simulink model "Offline_DataImport_AND_SCGAnalysis"  (R2020b)
settings: Solver=FixedStepDiscrete  StartTime=0.0  StopTime=param_sim_time  FixedStep=1/fs  MaxStep=1/fs  RelTol=1e-3
undefined symbols (not defined in the file): analyses, fs, param_tot_samples
libraries: dspstat3 x1
settings Model: PacingRate=100  Creator=rcord  LastModifiedBy=Rafael
settings SolverCC: ZeroCrossControl=DisableAll
settings DataIOCC: ExternalInput=[t, signals.scg.preprocessed_x, signals.scg.preprocessed_y, signals.scg.preprocessed_z]  LoadExternalInput=on  SignalLogging=off  DSMLogging=off  SaveTime=off  ReturnWorkspaceOutputs=off  TimeSaveName=t_preprocessing  OutputSaveName=out_SCGAnalysis  LoggingIntervals=[-inf,inf]
settings SFSimCC: CustomCodeUndefinedFunction=UseInterfaceOnly

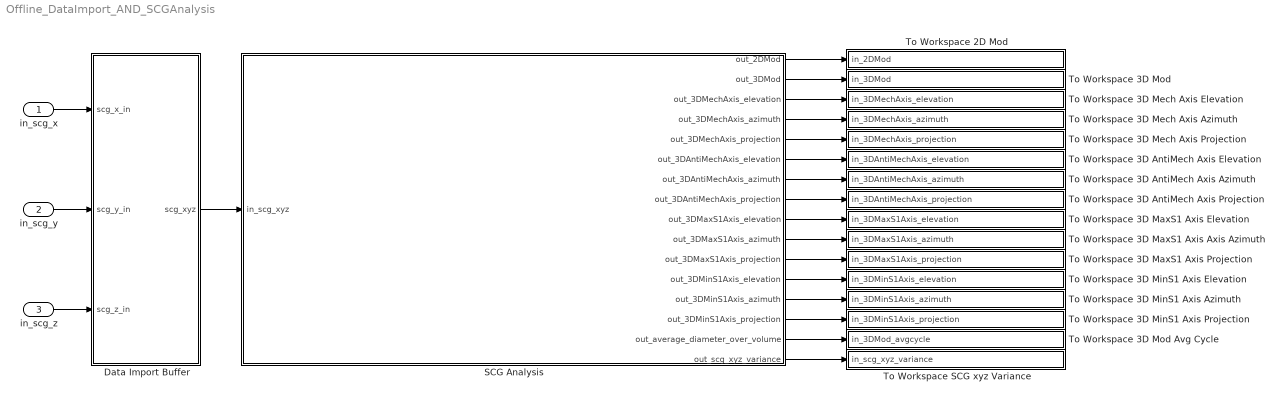
== system Offline_DataImport_AND_SCGAnalysis ==
  in_scg_x : Inport  SampleTime=1/fs
  in_scg_y : Inport  Port=2  SampleTime=1/fs
  in_scg_z : Inport  Port=3  SampleTime=1/fs
  Data Import Buffer : Subsystem
  SCG Analysis : Subsystem
      mask Display: image('C:\Users\Rafael\Dropbox\Post-Doc Research\SCG Analysis.png'); % Use "Edit Image" on toolstrip to change.
  To Workspace 2D Mod : Subsystem
      mask Display: disp('out_scg_analysis_2DMod')
  To Workspace 3D AntiMech Axis Azimuth : Subsystem
      mask Display: disp('out_scg_analysis_3DAntiMechAxis_azimuth')
  To Workspace 3D AntiMech Axis Elevation : Subsystem
      mask Display: disp('out_scg_analysis_3DAntiMechAxis_elevation')
  To Workspace 3D AntiMech Axis Projection : Subsystem
      mask Display: disp('out_scg_analysis_3DAntiMechAxis_projection')
  To Workspace 3D MaxS1 Axis Axis Azimuth : Subsystem
      mask Display: disp('out_scg_analysis_3DMaxS1Axis_azimuth')
  To Workspace 3D MaxS1 Axis Elevation : Subsystem
      mask Display: disp('out_scg_analysis_3DMaxS1Axis_elevation')
  To Workspace 3D MaxS1 Axis Projection : Subsystem
      mask Display: disp('out_scg_analysis_3DMaxS1Axis_projection')
  To Workspace 3D Mech Axis Azimuth : Subsystem
      mask Display: disp('out_scg_analysis_3DMechAxis_azimuth')
  To Workspace 3D Mech Axis Elevation : Subsystem
      mask Display: disp('out_scg_analysis_3DMechAxis_elevation')
  To Workspace 3D Mech Axis Projection : Subsystem
      mask Display: disp('out_scg_analysis_3DMechAxis_projection')
  To Workspace 3D MinS1 Axis Azimuth : Subsystem
      mask Display: disp('out_scg_analysis_3DMinS1Axis_azimuth')
  To Workspace 3D MinS1 Axis Elevation : Subsystem
      mask Display: disp('out_scg_analysis_3DMinS1Axis_elevation')
  To Workspace 3D MinS1 Axis Projection : Subsystem
      mask Display: disp('out_scg_analysis_3DMinS1Axis_projection')
  To Workspace 3D Mod : Subsystem
      mask Display: disp('out_scg_analysis_3DMod')
  To Workspace 3D Mod Avg Cycle : Subsystem
      mask Display: disp('out_scg_analysis_3DMod_avgcycle')
  To Workspace SCG xyz Variance : Subsystem
      mask Display: disp('out_scg_analysis_scg_xyz_variance')
  wires:
  in_scg_x/1 -> Data Import Buffer/1(scg_x_in)
  in_scg_y/1 -> Data Import Buffer/2(scg_y_in)
  in_scg_z/1 -> Data Import Buffer/3(scg_z_in)
  Data Import Buffer/1(scg_xyz) -> SCG Analysis/1(in_scg_xyz)
  SCG Analysis/16(out_scg_xyz_variance) -> To Workspace SCG xyz Variance/1(in_scg_xyz_variance)
  SCG Analysis/2(out_3DMod) -> To Workspace 3D Mod/1(in_3DMod)
  SCG Analysis/15(out_average_diameter_over_volume) -> To Workspace 3D Mod Avg Cycle/1(in_3DMod_avgcycle)
  SCG Analysis/1(out_2DMod) -> To Workspace 2D Mod/1(in_2DMod)
  SCG Analysis/3(out_3DMechAxis_elevation) -> To Workspace 3D Mech Axis Elevation/1(in_3DMechAxis_elevation)
  SCG Analysis/4(out_3DMechAxis_azimuth) -> To Workspace 3D Mech Axis Azimuth/1(in_3DMechAxis_azimuth)
  SCG Analysis/5(out_3DMechAxis_projection) -> To Workspace 3D Mech Axis Projection/1(in_3DMechAxis_projection)
  SCG Analysis/6(out_3DAntiMechAxis_elevation) -> To Workspace 3D AntiMech Axis Elevation/1(in_3DAntiMechAxis_elevation)
  SCG Analysis/7(out_3DAntiMechAxis_azimuth) -> To Workspace 3D AntiMech Axis Azimuth/1(in_3DAntiMechAxis_azimuth)
  SCG Analysis/8(out_3DAntiMechAxis_projection) -> To Workspace 3D AntiMech Axis Projection/1(in_3DAntiMechAxis_projection)
  SCG Analysis/9(out_3DMaxS1Axis_elevation) -> To Workspace 3D MaxS1 Axis Elevation/1(in_3DMaxS1Axis_elevation)
  SCG Analysis/10(out_3DMaxS1Axis_azimuth) -> To Workspace 3D MaxS1 Axis Axis Azimuth/1(in_3DMaxS1Axis_azimuth)
  SCG Analysis/11(out_3DMaxS1Axis_projection) -> To Workspace 3D MaxS1 Axis Projection/1(in_3DMaxS1Axis_projection)
  SCG Analysis/12(out_3DMinS1Axis_elevation) -> To Workspace 3D MinS1 Axis Elevation/1(in_3DMinS1Axis_elevation)
  SCG Analysis/13(out_3DMinS1Axis_azimuth) -> To Workspace 3D MinS1 Axis Azimuth/1(in_3DMinS1Axis_azimuth)
  SCG Analysis/14(out_3DMinS1Axis_projection) -> To Workspace 3D MinS1 Axis Projection/1(in_3DMinS1Axis_projection)

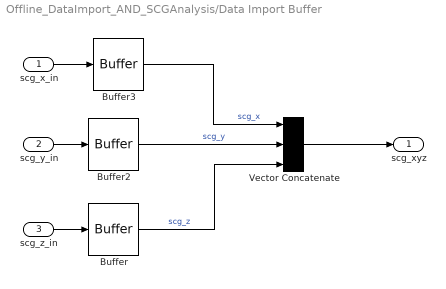
== system Offline_DataImport_AND_SCGAnalysis/Data Import Buffer ==
  scg_x_in : Inport
  scg_y_in : Inport  Port=2
  scg_z_in : Inport  Port=3
  Buffer : Buffer  N=param_tot_samples  OutputFrames=off
  Buffer2 : Buffer  N=param_tot_samples  OutputFrames=off
  Buffer3 : Buffer  N=param_tot_samples  OutputFrames=off
  Vector Concatenate : Concatenate  NumInputs=3  Mode=Multidimensional array  ConcatenateDimension=2
  scg_xyz : Outport  VectorParamsAs1DForOutWhenUnconnected=off
  wires:
  Buffer/1 -> Vector Concatenate/3  "scg_z"
  Buffer3/1 -> Vector Concatenate/1  "scg_x"
  scg_x_in/1 -> Buffer3/1
  Vector Concatenate/1 -> scg_xyz/1
  Buffer2/1 -> Vector Concatenate/2  "scg_y"
  scg_z_in/1 -> Buffer/1
  scg_y_in/1 -> Buffer2/1

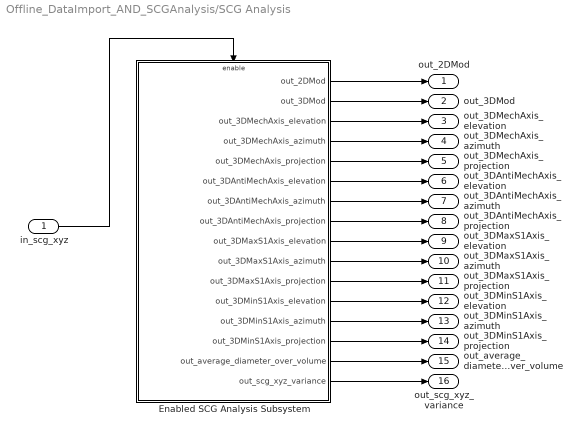
== system Offline_DataImport_AND_SCGAnalysis/SCG Analysis ==
  in_scg_xyz : Inport
  Enabled SCG Analysis Subsystem : Subsystem  TreatAsAtomicUnit=on
  out_2DMod : Outport  VectorParamsAs1DForOutWhenUnconnected=off
  out_3DMod : Outport  Port=2  VectorParamsAs1DForOutWhenUnconnected=off
  out_3DMechAxis_elevation : Outport  Port=3  VectorParamsAs1DForOutWhenUnconnected=off
  out_3DMechAxis_azimuth : Outport  Port=4  VectorParamsAs1DForOutWhenUnconnected=off
  out_3DMechAxis_projection : Outport  Port=5  VectorParamsAs1DForOutWhenUnconnected=off
  out_3DAntiMechAxis_elevation : Outport  Port=6  VectorParamsAs1DForOutWhenUnconnected=off
  out_3DAntiMechAxis_azimuth : Outport  Port=7  VectorParamsAs1DForOutWhenUnconnected=off
  out_3DAntiMechAxis_projection : Outport  Port=8  VectorParamsAs1DForOutWhenUnconnected=off
  out_3DMaxS1Axis_elevation : Outport  Port=9  VectorParamsAs1DForOutWhenUnconnected=off
  out_3DMaxS1Axis_azimuth : Outport  Port=10  VectorParamsAs1DForOutWhenUnconnected=off
  out_3DMaxS1Axis_projection : Outport  Port=11  VectorParamsAs1DForOutWhenUnconnected=off
  out_3DMinS1Axis_elevation : Outport  Port=12  VectorParamsAs1DForOutWhenUnconnected=off
  out_3DMinS1Axis_azimuth : Outport  Port=13  VectorParamsAs1DForOutWhenUnconnected=off
  out_3DMinS1Axis_projection : Outport  Port=14  VectorParamsAs1DForOutWhenUnconnected=off
  out_average_diameter_over_volume : Outport  Port=15  VectorParamsAs1DForOutWhenUnconnected=off
  out_scg_xyz_variance : Outport  Port=16  VectorParamsAs1DForOutWhenUnconnected=off
  wires:
  in_scg_xyz/1 -> Enabled SCG Analysis Subsystem/Enable
  Enabled SCG Analysis Subsystem/16(out_scg_xyz_variance) -> out_scg_xyz_variance/1
  Enabled SCG Analysis Subsystem/2(out_3DMod) -> out_3DMod/1
  Enabled SCG Analysis Subsystem/1(out_2DMod) -> out_2DMod/1
  Enabled SCG Analysis Subsystem/3(out_3DMechAxis_elevation) -> out_3DMechAxis_elevation/1
  Enabled SCG Analysis Subsystem/4(out_3DMechAxis_azimuth) -> out_3DMechAxis_azimuth/1
  Enabled SCG Analysis Subsystem/5(out_3DMechAxis_projection) -> out_3DMechAxis_projection/1
  Enabled SCG Analysis Subsystem/8(out_3DAntiMechAxis_projection) -> out_3DAntiMechAxis_projection/1
  Enabled SCG Analysis Subsystem/9(out_3DMaxS1Axis_elevation) -> out_3DMaxS1Axis_elevation/1
  Enabled SCG Analysis Subsystem/10(out_3DMaxS1Axis_azimuth) -> out_3DMaxS1Axis_azimuth/1
  Enabled SCG Analysis Subsystem/11(out_3DMaxS1Axis_projection) -> out_3DMaxS1Axis_projection/1
  Enabled SCG Analysis Subsystem/14(out_3DMinS1Axis_projection) -> out_3DMinS1Axis_projection/1
  Enabled SCG Analysis Subsystem/15(out_average_diameter_over_volume) -> out_average_diameter_over_volume/1
  Enabled SCG Analysis Subsystem/6(out_3DAntiMechAxis_elevation) -> out_3DAntiMechAxis_elevation/1
  Enabled SCG Analysis Subsystem/7(out_3DAntiMechAxis_azimuth) -> out_3DAntiMechAxis_azimuth/1
  Enabled SCG Analysis Subsystem/12(out_3DMinS1Axis_elevation) -> out_3DMinS1Axis_elevation/1
  Enabled SCG Analysis Subsystem/13(out_3DMinS1Axis_azimuth) -> out_3DMinS1Axis_azimuth/1

== system Offline_DataImport_AND_SCGAnalysis/To Workspace 2D Mod ==
  in_2DMod : Inport
  Enabled To Workspace 2DMod Subsystem : Subsystem  TreatAsAtomicUnit=on
  wires:
  in_2DMod/1 -> Enabled To Workspace 2DMod Subsystem/Enable

== system Offline_DataImport_AND_SCGAnalysis/To Workspace 3D AntiMech Axis Azimuth ==
  in_3DAntiMechAxis_azimuth : Inport
  Enabled To Workspace 3DAntiMechAxis Azimuth : Subsystem  TreatAsAtomicUnit=on
  wires:
  in_3DAntiMechAxis_azimuth/1 -> Enabled To Workspace 3DAntiMechAxis Azimuth/Enable

== system Offline_DataImport_AND_SCGAnalysis/To Workspace 3D AntiMech Axis Elevation ==
  in_3DAntiMechAxis_elevation : Inport
  Enabled To Workspace 3DAntiMechAxis Elevation : Subsystem  TreatAsAtomicUnit=on
  wires:
  in_3DAntiMechAxis_elevation/1 -> Enabled To Workspace 3DAntiMechAxis Elevation/Enable

== system Offline_DataImport_AND_SCGAnalysis/To Workspace 3D AntiMech Axis Projection ==
  in_3DAntiMechAxis_projection : Inport
  Enabled To Workspace 3DAntiMechAxis Projection : Subsystem  TreatAsAtomicUnit=on
  wires:
  in_3DAntiMechAxis_projection/1 -> Enabled To Workspace 3DAntiMechAxis Projection/Enable

== system Offline_DataImport_AND_SCGAnalysis/To Workspace 3D MaxS1 Axis Axis Azimuth ==
  in_3DMaxS1Axis_azimuth : Inport
  Enabled To Workspace 3DMaxS1Axis Azimuth : Subsystem  TreatAsAtomicUnit=on
  wires:
  in_3DMaxS1Axis_azimuth/1 -> Enabled To Workspace 3DMaxS1Axis Azimuth/Enable

== system Offline_DataImport_AND_SCGAnalysis/To Workspace 3D MaxS1 Axis Elevation ==
  in_3DMaxS1Axis_elevation : Inport
  Enabled To Workspace 3DMaxS1Axis Elevation : Subsystem  TreatAsAtomicUnit=on
  wires:
  in_3DMaxS1Axis_elevation/1 -> Enabled To Workspace 3DMaxS1Axis Elevation/Enable

== system Offline_DataImport_AND_SCGAnalysis/To Workspace 3D MaxS1 Axis Projection ==
  in_3DMaxS1Axis_projection : Inport
  Enabled To Workspace 3DMaxS1Axis Projection : Subsystem  TreatAsAtomicUnit=on
  wires:
  in_3DMaxS1Axis_projection/1 -> Enabled To Workspace 3DMaxS1Axis Projection/Enable

== system Offline_DataImport_AND_SCGAnalysis/To Workspace 3D Mech Axis Azimuth ==
  in_3DMechAxis_azimuth : Inport
  Enabled To Workspace 3DMechAxis Azimuth : Subsystem  TreatAsAtomicUnit=on
  wires:
  in_3DMechAxis_azimuth/1 -> Enabled To Workspace 3DMechAxis Azimuth/Enable

== system Offline_DataImport_AND_SCGAnalysis/To Workspace 3D Mech Axis Elevation ==
  in_3DMechAxis_elevation : Inport
  Enabled To Workspace 3DMechAxis Elevation : Subsystem  TreatAsAtomicUnit=on
  wires:
  in_3DMechAxis_elevation/1 -> Enabled To Workspace 3DMechAxis Elevation/Enable

== system Offline_DataImport_AND_SCGAnalysis/To Workspace 3D Mech Axis Projection ==
  in_3DMechAxis_projection : Inport
  Enabled To Workspace 3DMechAxis Projection : Subsystem  TreatAsAtomicUnit=on
  wires:
  in_3DMechAxis_projection/1 -> Enabled To Workspace 3DMechAxis Projection/Enable

== system Offline_DataImport_AND_SCGAnalysis/To Workspace 3D MinS1 Axis Azimuth ==
  in_3DMinS1Axis_azimuth : Inport
  Enabled To Workspace 3DMinS1Axis Azimuth : Subsystem  TreatAsAtomicUnit=on
  wires:
  in_3DMinS1Axis_azimuth/1 -> Enabled To Workspace 3DMinS1Axis Azimuth/Enable

== system Offline_DataImport_AND_SCGAnalysis/To Workspace 3D MinS1 Axis Elevation ==
  in_3DMinS1Axis_elevation : Inport
  Enabled To Workspace 3DMinS1Axis Elevation : Subsystem  TreatAsAtomicUnit=on
  wires:
  in_3DMinS1Axis_elevation/1 -> Enabled To Workspace 3DMinS1Axis Elevation/Enable

== system Offline_DataImport_AND_SCGAnalysis/To Workspace 3D MinS1 Axis Projection ==
  in_3DMinS1Axis_projection : Inport
  Enabled To Workspace 3DMinS1Axis Projection : Subsystem  TreatAsAtomicUnit=on
  wires:
  in_3DMinS1Axis_projection/1 -> Enabled To Workspace 3DMinS1Axis Projection/Enable

== system Offline_DataImport_AND_SCGAnalysis/To Workspace 3D Mod ==
  in_3DMod : Inport
  Enabled To Workspace 3DMod Subsystem : Subsystem  TreatAsAtomicUnit=on
  wires:
  in_3DMod/1 -> Enabled To Workspace 3DMod Subsystem/Enable

== system Offline_DataImport_AND_SCGAnalysis/To Workspace 3D Mod Avg Cycle ==
  in_3DMod_avgcycle : Inport
  Enabled To Workspace 3DMod Avg Cycle Subsystem : Subsystem  TreatAsAtomicUnit=on
  wires:
  in_3DMod_avgcycle/1 -> Enabled To Workspace 3DMod Avg Cycle Subsystem/Enable

== system Offline_DataImport_AND_SCGAnalysis/To Workspace SCG xyz Variance ==
  in_scg_xyz_variance : Inport
  Enabled To Workspace SCG xyz Variance Subsystem : Subsystem  TreatAsAtomicUnit=on
  wires:
  in_scg_xyz_variance/1 -> Enabled To Workspace SCG xyz Variance Subsystem/Enable

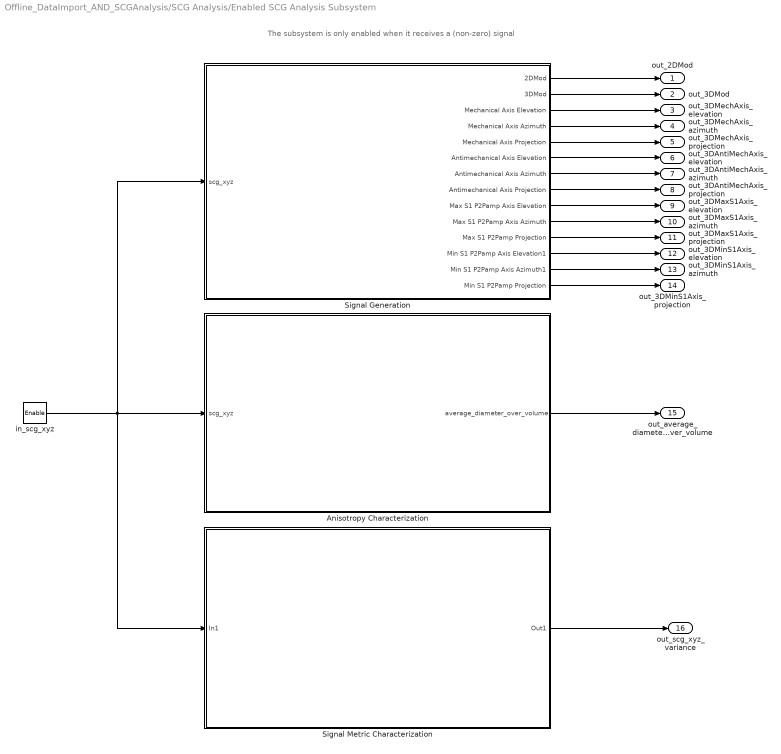
== system Offline_DataImport_AND_SCGAnalysis/SCG Analysis/Enabled SCG Analysis Subsystem ==
  note: The subsystem is only enabled when it receives a (non-zero) signal
  in_scg_xyz : EnablePort  PropagateVarSize=During execution  ShowOutputPort=on
  Anisotropy Characterization : Subsystem
      mask Display: image('C:\Users\Rafael\Dropbox\Post-Doc Research\Anisotropy.png'); % Use "Edit Image" on toolstrip to change.
  Signal Generation : Subsystem
      mask Display: image('C:\Users\Rafael\Dropbox\Post-Doc Research\Signal Generation.png'); % Use "Edit Image" on toolstrip to change.
  Signal Metric Characterization : Subsystem
      mask Display: image('C:\Users\Rafael\Dropbox\Post-Doc Research\SCGAnalysisSymbol.jpg'); % Use "Edit Image" on toolstrip to change.
  out_2DMod : Outport  VectorParamsAs1DForOutWhenUnconnected=off
  out_3DMod : Outport  Port=2  VectorParamsAs1DForOutWhenUnconnected=off
  out_3DMechAxis_elevation : Outport  Port=3  VectorParamsAs1DForOutWhenUnconnected=off
  out_3DMechAxis_azimuth : Outport  Port=4  VectorParamsAs1DForOutWhenUnconnected=off
  out_3DMechAxis_projection : Outport  Port=5  VectorParamsAs1DForOutWhenUnconnected=off
  out_3DAntiMechAxis_elevation : Outport  Port=6  VectorParamsAs1DForOutWhenUnconnected=off
  out_3DAntiMechAxis_azimuth : Outport  Port=7  VectorParamsAs1DForOutWhenUnconnected=off
  out_3DAntiMechAxis_projection : Outport  Port=8  VectorParamsAs1DForOutWhenUnconnected=off
  out_3DMaxS1Axis_elevation : Outport  Port=9  VectorParamsAs1DForOutWhenUnconnected=off
  out_3DMaxS1Axis_azimuth : Outport  Port=10  VectorParamsAs1DForOutWhenUnconnected=off
  out_3DMaxS1Axis_projection : Outport  Port=11  VectorParamsAs1DForOutWhenUnconnected=off
  out_3DMinS1Axis_elevation : Outport  Port=12  VectorParamsAs1DForOutWhenUnconnected=off
  out_3DMinS1Axis_azimuth : Outport  Port=13  VectorParamsAs1DForOutWhenUnconnected=off
  out_3DMinS1Axis_projection : Outport  Port=14  VectorParamsAs1DForOutWhenUnconnected=off
  out_average_diameter_over_volume : Outport  Port=15  VectorParamsAs1DForOutWhenUnconnected=off
  out_scg_xyz_variance : Outport  Port=16  VectorParamsAs1DForOutWhenUnconnected=off
  wires:
  in_scg_xyz/1 -> Anisotropy Characterization/1(scg_xyz), Signal Metric Characterization/1(In1), Signal Generation/1(scg_xyz)
  Signal Generation/1(2DMod) -> out_2DMod/1
  Signal Generation/2(3DMod) -> out_3DMod/1
  Signal Generation/5(Mechanical Axis Projection) -> out_3DMechAxis_projection/1
  Signal Generation/8(Antimechanical Axis Projection) -> out_3DAntiMechAxis_projection/1
  Signal Generation/11(Max S1 P2Pamp Projection) -> out_3DMaxS1Axis_projection/1
  Signal Generation/14(Min S1 P2Pamp Projection) -> out_3DMinS1Axis_projection/1
  Signal Metric Characterization/1(Out1) -> out_scg_xyz_variance/1
  Signal Generation/3(Mechanical Axis Elevation) -> out_3DMechAxis_elevation/1
  Signal Generation/4(Mechanical Axis Azimuth) -> out_3DMechAxis_azimuth/1
  Signal Generation/9(Max S1 P2Pamp Axis Elevation) -> out_3DMaxS1Axis_elevation/1
  Signal Generation/10(Max S1 P2Pamp Axis Azimuth) -> out_3DMaxS1Axis_azimuth/1
  Anisotropy Characterization/1(average_diameter_over_volume) -> out_average_diameter_over_volume/1
  Signal Generation/6(Antimechanical Axis Elevation) -> out_3DAntiMechAxis_elevation/1
  Signal Generation/7(Antimechanical Axis Azimuth) -> out_3DAntiMechAxis_azimuth/1
  Signal Generation/12(Min S1 P2Pamp Axis Elevation1) -> out_3DMinS1Axis_elevation/1
  Signal Generation/13(Min S1 P2Pamp Axis Azimuth1) -> out_3DMinS1Axis_azimuth/1

== system Offline_DataImport_AND_SCGAnalysis/To Workspace 2D Mod/Enabled To Workspace 2DMod Subsystem ==
  Enable : EnablePort  PropagateVarSize=During execution  ShowOutputPort=on
  To Workspace SCG 2DMod : ToWorkspace  VariableName=out_scg_analysis_2DMod  SaveFormat=Structure  SampleTime=-1
  wires:
  Enable/1 -> To Workspace SCG 2DMod/1

== system Offline_DataImport_AND_SCGAnalysis/To Workspace 3D AntiMech Axis Azimuth/Enabled To Workspace 3DAntiMechAxis Azimuth ==
  Enable : EnablePort  PropagateVarSize=During execution  ShowOutputPort=on
  To Workspace SCG 3DAntiMechAxis Azimuth : ToWorkspace  VariableName=out_scg_analysis_3DAntiMechAxis_azimuth  SaveFormat=Structure  SampleTime=-1
  wires:
  Enable/1 -> To Workspace SCG 3DAntiMechAxis Azimuth/1

== system Offline_DataImport_AND_SCGAnalysis/To Workspace 3D AntiMech Axis Elevation/Enabled To Workspace 3DAntiMechAxis Elevation ==
  Enable : EnablePort  PropagateVarSize=During execution  ShowOutputPort=on
  To Workspace SCG 3DAntiMechAxis Elevation : ToWorkspace  VariableName=out_scg_analysis_3DAntiMechAxis_elevation  SaveFormat=Structure  SampleTime=-1
  wires:
  Enable/1 -> To Workspace SCG 3DAntiMechAxis Elevation/1

== system Offline_DataImport_AND_SCGAnalysis/To Workspace 3D AntiMech Axis Projection/Enabled To Workspace 3DAntiMechAxis Projection ==
  Enable : EnablePort  PropagateVarSize=During execution  ShowOutputPort=on
  To Workspace SCG 3DAntiMechAxis Projection : ToWorkspace  VariableName=out_scg_analysis_3DAntiMechAxis_projection  SaveFormat=Structure  SampleTime=-1
  wires:
  Enable/1 -> To Workspace SCG 3DAntiMechAxis Projection/1

== system Offline_DataImport_AND_SCGAnalysis/To Workspace 3D MaxS1 Axis Axis Azimuth/Enabled To Workspace 3DMaxS1Axis Azimuth ==
  Enable : EnablePort  PropagateVarSize=During execution  ShowOutputPort=on
  To Workspace SCG 3DMaxS1Axis Azimuth : ToWorkspace  VariableName=out_scg_analysis_3DMaxS1Axis_azimuth  SaveFormat=Structure  SampleTime=-1
  wires:
  Enable/1 -> To Workspace SCG 3DMaxS1Axis Azimuth/1

== system Offline_DataImport_AND_SCGAnalysis/To Workspace 3D MaxS1 Axis Elevation/Enabled To Workspace 3DMaxS1Axis Elevation ==
  Enable : EnablePort  PropagateVarSize=During execution  ShowOutputPort=on
  To Workspace SCG 3DMaxS1Axis Elevation : ToWorkspace  VariableName=out_scg_analysis_3DMaxS1Axis_elevation  SaveFormat=Structure  SampleTime=-1
  wires:
  Enable/1 -> To Workspace SCG 3DMaxS1Axis Elevation/1

== system Offline_DataImport_AND_SCGAnalysis/To Workspace 3D MaxS1 Axis Projection/Enabled To Workspace 3DMaxS1Axis Projection ==
  Enable : EnablePort  PropagateVarSize=During execution  ShowOutputPort=on
  To Workspace SCG 3DMaxS1Axis Projection : ToWorkspace  VariableName=out_scg_analysis_3DMaxS1Axis_projection  SaveFormat=Structure  SampleTime=-1
  wires:
  Enable/1 -> To Workspace SCG 3DMaxS1Axis Projection/1

== system Offline_DataImport_AND_SCGAnalysis/To Workspace 3D Mech Axis Azimuth/Enabled To Workspace 3DMechAxis Azimuth ==
  Enable : EnablePort  PropagateVarSize=During execution  ShowOutputPort=on
  To Workspace SCG 3DMechAxis Azimuth : ToWorkspace  VariableName=out_scg_analysis_3DMechAxis_azimuth  SaveFormat=Structure  SampleTime=-1
  wires:
  Enable/1 -> To Workspace SCG 3DMechAxis Azimuth/1

== system Offline_DataImport_AND_SCGAnalysis/To Workspace 3D Mech Axis Elevation/Enabled To Workspace 3DMechAxis Elevation ==
  Enable : EnablePort  PropagateVarSize=During execution  ShowOutputPort=on
  To Workspace SCG 3DMechAxis Elevation : ToWorkspace  VariableName=out_scg_analysis_3DMechAxis_elevation  SaveFormat=Structure  SampleTime=-1
  wires:
  Enable/1 -> To Workspace SCG 3DMechAxis Elevation/1

== system Offline_DataImport_AND_SCGAnalysis/To Workspace 3D Mech Axis Projection/Enabled To Workspace 3DMechAxis Projection ==
  Enable : EnablePort  PropagateVarSize=During execution  ShowOutputPort=on
  To Workspace SCG 3DMechAxis Projection : ToWorkspace  VariableName=out_scg_analysis_3DMechAxis_projection  SaveFormat=Structure  SampleTime=-1
  wires:
  Enable/1 -> To Workspace SCG 3DMechAxis Projection/1

== system Offline_DataImport_AND_SCGAnalysis/To Workspace 3D MinS1 Axis Azimuth/Enabled To Workspace 3DMinS1Axis Azimuth ==
  Enable : EnablePort  PropagateVarSize=During execution  ShowOutputPort=on
  To Workspace SCG 3DMinS1Axis Azimuth : ToWorkspace  VariableName=out_scg_analysis_3DMinS1Axis_azimuth  SaveFormat=Structure  SampleTime=-1
  wires:
  Enable/1 -> To Workspace SCG 3DMinS1Axis Azimuth/1

== system Offline_DataImport_AND_SCGAnalysis/To Workspace 3D MinS1 Axis Elevation/Enabled To Workspace 3DMinS1Axis Elevation ==
  Enable : EnablePort  PropagateVarSize=During execution  ShowOutputPort=on
  To Workspace SCG 3DMinS1Axis Elevation : ToWorkspace  VariableName=out_scg_analysis_3DMinS1Axis_elevation  SaveFormat=Structure  SampleTime=-1
  wires:
  Enable/1 -> To Workspace SCG 3DMinS1Axis Elevation/1

== system Offline_DataImport_AND_SCGAnalysis/To Workspace 3D MinS1 Axis Projection/Enabled To Workspace 3DMinS1Axis Projection ==
  Enable : EnablePort  PropagateVarSize=During execution  ShowOutputPort=on
  To Workspace SCG 3DMinS1Axis Projection : ToWorkspace  VariableName=out_scg_analysis_3DMinS1Axis_projection  SaveFormat=Structure  SampleTime=-1
  wires:
  Enable/1 -> To Workspace SCG 3DMinS1Axis Projection/1

== system Offline_DataImport_AND_SCGAnalysis/To Workspace 3D Mod/Enabled To Workspace 3DMod Subsystem ==
  Enable : EnablePort  PropagateVarSize=During execution  ShowOutputPort=on
  To Workspace SCG 3DMod : ToWorkspace  VariableName=out_scg_analysis_3DMod  SaveFormat=Structure  SampleTime=-1
  wires:
  Enable/1 -> To Workspace SCG 3DMod/1

== system Offline_DataImport_AND_SCGAnalysis/To Workspace 3D Mod Avg Cycle/Enabled To Workspace 3DMod Avg Cycle Subsystem ==
  Enable : EnablePort  ShowOutputPort=on
  To Workspace SCG 3DMod Avg Cycle : ToWorkspace  VariableName=out_scg_analysis_3DMod_avgcycle  SaveFormat=Structure  SampleTime=-1
  wires:
  Enable/1 -> To Workspace SCG 3DMod Avg Cycle/1

== system Offline_DataImport_AND_SCGAnalysis/To Workspace SCG xyz Variance/Enabled To Workspace SCG xyz Variance Subsystem ==
  note: The subsystem is only enabled when it receives a (non-zero) signal
  Enable : EnablePort  PropagateVarSize=During execution  ShowOutputPort=on
  To Workspace SCG xyz variance : ToWorkspace  VariableName=out_scg_analysis_scg_xyz_variance  SaveFormat=Structure  SampleTime=-1
      settings: MaxDataPoints=3
  wires:
  Enable/1 -> To Workspace SCG xyz variance/1

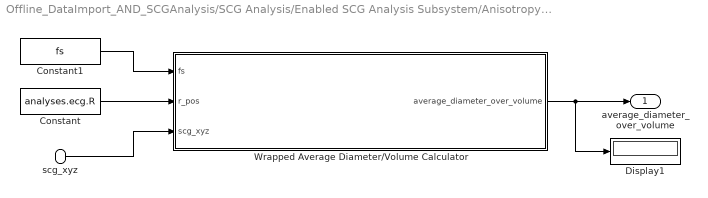
== system Offline_DataImport_AND_SCGAnalysis/SCG Analysis/Enabled SCG Analysis Subsystem/Anisotropy Characterization ==
  scg_xyz : Inport
  Constant : Constant  Value=analyses.ecg.R
  Constant1 : Constant  Value=fs
  Display1 : Display
  Wrapped Average Diameter/Volume Calculator : MATLAB Function  TreatAsAtomicUnit=on
  average_diameter_over_volume : Outport
  wires:
  Constant/1 -> Wrapped Average Diameter/Volume Calculator/2(r_pos)
  scg_xyz/1 -> Wrapped Average Diameter/Volume Calculator/3(scg_xyz)
  Constant1/1 -> Wrapped Average Diameter/Volume Calculator/1(fs)
  Wrapped Average Diameter/Volume Calculator/1(average_diameter_over_volume) -> average_diameter_over_volume/1, Display1/1

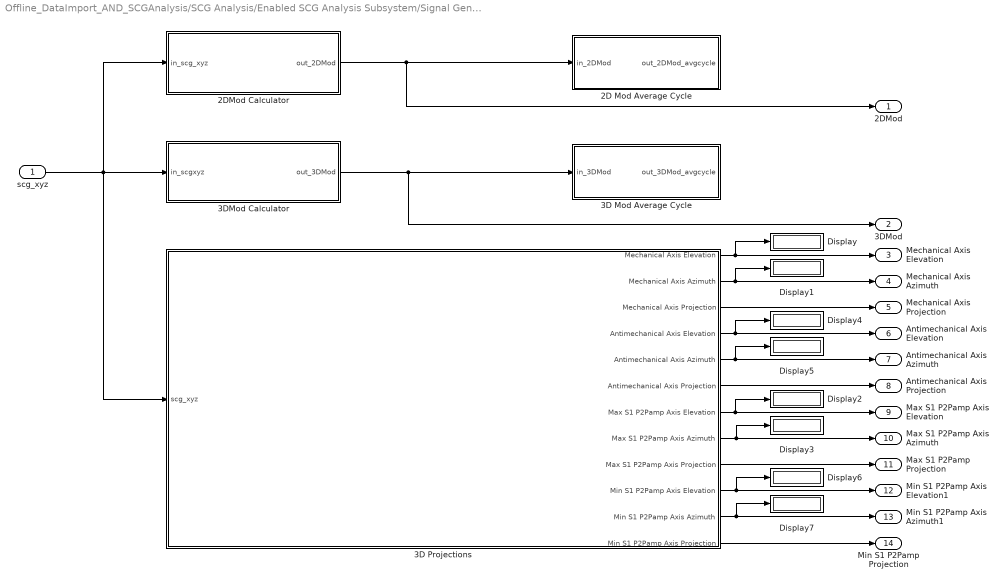
== system Offline_DataImport_AND_SCGAnalysis/SCG Analysis/Enabled SCG Analysis Subsystem/Signal Generation ==
  scg_xyz : Inport
  2D Mod Average Cycle : Subsystem
  2DMod Calculator : Subsystem  mask{xyz2Dcombo=xz (transverse plane)}
      mask prompts: xyz2Dcombo "2D component combination:"
      mask init:
      | if xyz2Dcombo == 1
      |     param_2Dxyzcombo = 'xy';
      | elseif xyz2Dcombo == 2
      |     param_2Dxyzcombo = 'yz';
      | elseif xyz2Dcombo == 3
      |     param_2Dxyzcombo = 'xz';
      | end
      | 
      | assignin('base','param_2Dxyzcombo', param_2Dxyzcombo)
      mask TypeOptions xyz2Dcombo: xy (coronal plane) | yz (sagittal plane) | xz (transverse plane)
      mask DialogControl DescGroupVar Prompt: 2D Modulus Calculator
      mask DialogControl DescTextVar Prompt: Subsystem to calculate a 2D modulus signal from a user-specified combination of any two of the SCG x, y, or z components.
  3D Mod Average Cycle : Subsystem
  3D Projections : Subsystem
      mask Display: image('C:\Users\Rafael\Dropbox\Post-Doc Research\Coordinate Frames.png'); % Use "Edit Image" on toolstrip to change.
  3DMod Calculator : Subsystem
  Display{,1..7} (8 alike) : Display
  2DMod : Outport
  3DMod : Outport  Port=2
  Mechanical Axis Elevation : Outport  Port=3
  Mechanical Axis Azimuth : Outport  Port=4
  Mechanical Axis Projection : Outport  Port=5
  Antimechanical Axis Elevation : Outport  Port=6
  Antimechanical Axis Azimuth : Outport  Port=7
  Antimechanical Axis Projection : Outport  Port=8
  Max S1 P2Pamp Axis Elevation : Outport  Port=9
  Max S1 P2Pamp Axis Azimuth : Outport  Port=10
  Max S1 P2Pamp Projection : Outport  Port=11
  Min S1 P2Pamp Axis Elevation1 : Outport  Port=12
  Min S1 P2Pamp Axis Azimuth1 : Outport  Port=13
  Min S1 P2Pamp Projection : Outport  Port=14
  wires:
  3D Projections/1(Mechanical Axis Elevation) -> Mechanical Axis Elevation/1, Display/1
  3D Projections/7(Max S1 P2Pamp Axis Elevation) -> Max S1 P2Pamp Axis Elevation/1, Display2/1
  3DMod Calculator/1(out_3DMod) -> 3D Mod Average Cycle/1(in_3DMod), 3DMod/1
  3D Projections/8(Max S1 P2Pamp Axis Azimuth) -> Max S1 P2Pamp Axis Azimuth/1, Display3/1
  3D Projections/9(Max S1 P2Pamp Axis Projection) -> Max S1 P2Pamp Projection/1
  3D Projections/12(Min S1 P2Pamp Axis Projection) -> Min S1 P2Pamp Projection/1
  3D Projections/2(Mechanical Axis Azimuth) -> Mechanical Axis Azimuth/1, Display1/1
  2DMod Calculator/1(out_2DMod) -> 2D Mod Average Cycle/1(in_2DMod), 2DMod/1
  scg_xyz/1 -> 3DMod Calculator/1(in_scgxyz), 2DMod Calculator/1(in_scg_xyz), 3D Projections/1(scg_xyz)
  3D Projections/3(Mechanical Axis Projection) -> Mechanical Axis Projection/1
  3D Projections/6(Antimechanical Axis Projection) -> Antimechanical Axis Projection/1
  3D Projections/4(Antimechanical Axis Elevation) -> Display4/1, Antimechanical Axis Elevation/1
  3D Projections/5(Antimechanical Axis Azimuth) -> Display5/1, Antimechanical Axis Azimuth/1
  3D Projections/10(Min S1 P2Pamp Axis Elevation) -> Display6/1, Min S1 P2Pamp Axis Elevation1/1
  3D Projections/11(Min S1 P2Pamp Axis Azimuth) -> Display7/1, Min S1 P2Pamp Axis Azimuth1/1

== system Offline_DataImport_AND_SCGAnalysis/SCG Analysis/Enabled SCG Analysis Subsystem/Signal Metric Characterization ==
  In1 : Inport
  SCG xyz Variance : Display
  Variance : dspstat3/Variance  run=off  InputProcessing=Columns as channels (frame based)  reset_popup=None  directionMode=Each column  dimension=1  roiEnable=off  roiType=Rectangles  roiPortion=Entire ROI  roiOutput=Individual statistics for each ROI  roiFlag=off  roundingMode=Floor  overflowMode=off
  Out1 : Outport
  wires:
  Variance/1 -> Out1/1, SCG xyz Variance/1
  In1/1 -> Variance/1

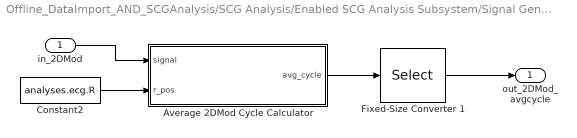
== system Offline_DataImport_AND_SCGAnalysis/SCG Analysis/Enabled SCG Analysis Subsystem/Signal Generation/2D Mod Average Cycle ==
  in_2DMod : Inport
  Average 2DMod Cycle Calculator : MATLAB Function  TreatAsAtomicUnit=on
  Constant2 : Constant  Value=analyses.ecg.R
  Fixed-Size Converter 1 : Selector  NumberOfDimensions=2  IndexOptions=Index vector (dialog),Index vector (dialog)  Indices=[1:min(analyses.ecg.RR)],1  OutputSizes=1,1
  out_2DMod_avgcycle : Outport  VectorParamsAs1DForOutWhenUnconnected=off
  wires:
  Constant2/1 -> Average 2DMod Cycle Calculator/2(r_pos)
  Average 2DMod Cycle Calculator/1(avg_cycle) -> Fixed-Size Converter 1/1
  in_2DMod/1 -> Average 2DMod Cycle Calculator/1(signal)
  Fixed-Size Converter 1/1 -> out_2DMod_avgcycle/1

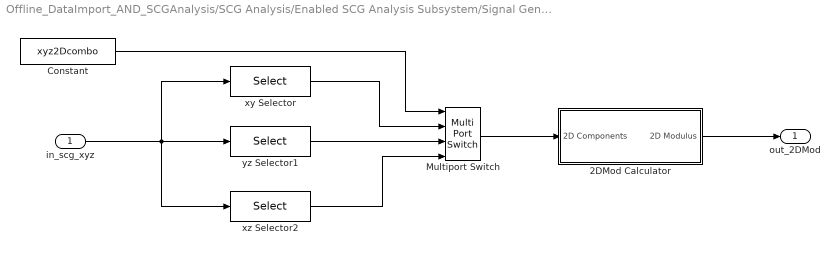
== system Offline_DataImport_AND_SCGAnalysis/SCG Analysis/Enabled SCG Analysis Subsystem/Signal Generation/2DMod Calculator ==
  in_scg_xyz : Inport
  2DMod Calculator : Subsystem
  Constant : Constant  Value=xyz2Dcombo
  Multiport Switch : MultiPortSwitch
  xy Selector : Selector  NumberOfDimensions=2  IndexOptions=Select all,Index vector (dialog)  Indices=[1:min(analyses.ecg.RR)],[1 2]  OutputSizes=1,1
  xz Selector2 : Selector  NumberOfDimensions=2  IndexOptions=Select all,Index vector (dialog)  Indices=[1:min(analyses.ecg.RR)],[1 3]  OutputSizes=1,1
  yz Selector1 : Selector  NumberOfDimensions=2  IndexOptions=Select all,Index vector (dialog)  Indices=[1:min(analyses.ecg.RR)],[2 3]  OutputSizes=1,1
  out_2DMod : Outport  VectorParamsAs1DForOutWhenUnconnected=off
  wires:
  2DMod Calculator/1(2D Modulus) -> out_2DMod/1
  in_scg_xyz/1 -> xz Selector2/1, xy Selector/1, yz Selector1/1
  Constant/1 -> Multiport Switch/1
  Multiport Switch/1 -> 2DMod Calculator/1(2D Components)
  xy Selector/1 -> Multiport Switch/2
  yz Selector1/1 -> Multiport Switch/3
  xz Selector2/1 -> Multiport Switch/4

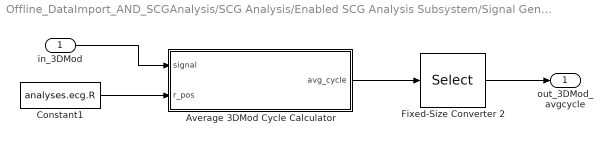
== system Offline_DataImport_AND_SCGAnalysis/SCG Analysis/Enabled SCG Analysis Subsystem/Signal Generation/3D Mod Average Cycle ==
  in_3DMod : Inport
  Average 3DMod Cycle Calculator : MATLAB Function  TreatAsAtomicUnit=on
  Constant1 : Constant  Value=analyses.ecg.R
  Fixed-Size Converter 2 : Selector  NumberOfDimensions=2  IndexOptions=Index vector (dialog),Index vector (dialog)  Indices=[1:min(analyses.ecg.RR)],1  OutputSizes=1,1
  out_3DMod_avgcycle : Outport  VectorParamsAs1DForOutWhenUnconnected=off
  wires:
  Average 3DMod Cycle Calculator/1(avg_cycle) -> Fixed-Size Converter 2/1
  Fixed-Size Converter 2/1 -> out_3DMod_avgcycle/1
  Constant1/1 -> Average 3DMod Cycle Calculator/2(r_pos)
  in_3DMod/1 -> Average 3DMod Cycle Calculator/1(signal)

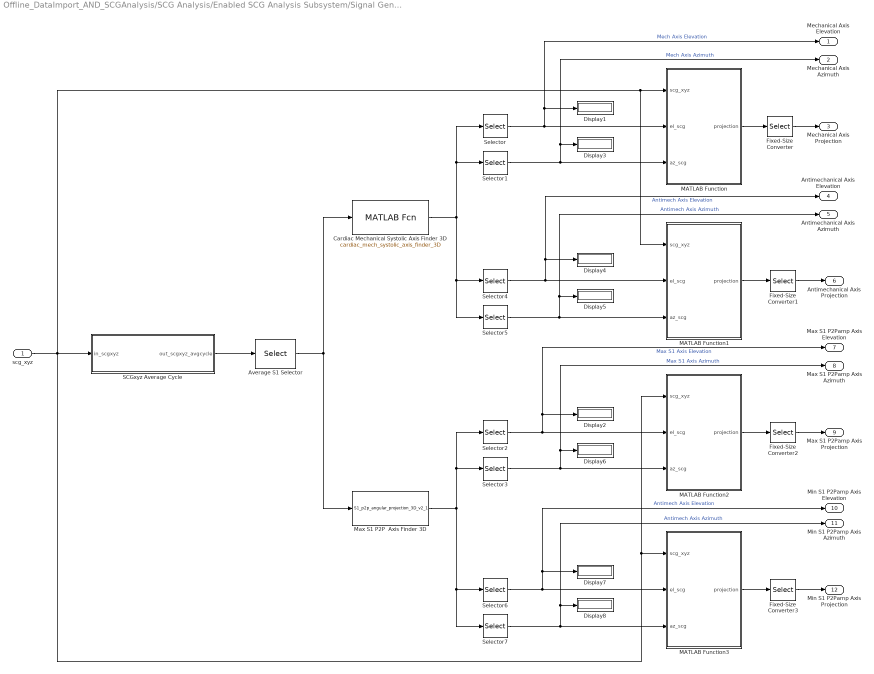
== system Offline_DataImport_AND_SCGAnalysis/SCG Analysis/Enabled SCG Analysis Subsystem/Signal Generation/3D Projections ==
  scg_xyz : Inport
  Average S1 Selector : Selector  NumberOfDimensions=2  InputPortWidth=3  IndexOptions=Index vector (dialog),Index vector (dialog)  Indices=[1:fs*0.2],[1 2 3]  OutputSizes=1,1
  Cardiac Mechanical Systolic Axis Finder 3D : MATLABFcn  MATLABFcn=cardiac_mech_systolic_axis_finder_3D  OutputDimensions=4  Output1D=off
  Display{1..8} (8 alike) : Display
  Fixed-Size Converter{,1..3} (4 alike) : Selector  NumberOfDimensions=2  IndexOptions=Index vector (dialog),Index vector (dialog)  Indices=1,[1:param_tot_samples]  OutputSizes=1,1
  MATLAB Function : MATLAB Function  TreatAsAtomicUnit=on
  MATLAB Function1 : MATLAB Function  TreatAsAtomicUnit=on
  MATLAB Function2 : MATLAB Function  TreatAsAtomicUnit=on
  MATLAB Function3 : MATLAB Function  TreatAsAtomicUnit=on
  Max S1 P2P  Axis Finder 3D : MATLABFcn  MATLABFcn=S1_p2p_angular_projection_3D_v2_1  OutputDimensions=4  Output1D=off
  SCGxyz Average Cycle : Subsystem
  Selector : Selector  InputPortWidth=4  IndexOptions=Index vector (dialog)  Indices=[1]  OutputSizes=1
  Selector1 : Selector  InputPortWidth=4  IndexOptions=Index vector (dialog)  Indices=[2]  OutputSizes=1
  Selector2 : Selector  InputPortWidth=4  IndexOptions=Index vector (dialog)  Indices=[1]  OutputSizes=1
  Selector3 : Selector  InputPortWidth=4  IndexOptions=Index vector (dialog)  Indices=[2]  OutputSizes=1
  Selector4 : Selector  InputPortWidth=4  IndexOptions=Index vector (dialog)  Indices=[3]  OutputSizes=1
  Selector5 : Selector  InputPortWidth=4  IndexOptions=Index vector (dialog)  Indices=[4]  OutputSizes=1
  Selector6 : Selector  InputPortWidth=4  IndexOptions=Index vector (dialog)  Indices=[3]  OutputSizes=1
  Selector7 : Selector  InputPortWidth=4  IndexOptions=Index vector (dialog)  Indices=[4]  OutputSizes=1
  Mechanical Axis Elevation : Outport
  Mechanical Axis Azimuth : Outport  Port=2
  Mechanical Axis Projection : Outport  Port=3
  Antimechanical Axis Elevation : Outport  Port=4
  Antimechanical Axis Azimuth : Outport  Port=5
  Antimechanical Axis Projection : Outport  Port=6
  Max S1 P2Pamp Axis Elevation : Outport  Port=7
  Max S1 P2Pamp Axis Azimuth : Outport  Port=8
  Max S1 P2Pamp Axis Projection : Outport  Port=9
  Min S1 P2Pamp Axis Elevation : Outport  Port=10
  Min S1 P2Pamp Axis Azimuth : Outport  Port=11
  Min S1 P2Pamp Axis Projection : Outport  Port=12
  wires:
  scg_xyz/1 -> MATLAB Function1/1(scg_xyz), MATLAB Function/1(scg_xyz), MATLAB Function2/1(scg_xyz), MATLAB Function3/1(scg_xyz), SCGxyz Average Cycle/1(in_scgxyz)
  Selector4/1 -> MATLAB Function1/2(el_scg), Antimechanical Axis Elevation/1, Display4/1  "Antimech Axis Elevation"
  Selector2/1 -> MATLAB Function2/2(el_scg), Max S1 P2Pamp Axis Elevation/1, Display2/1  "Max S1 Axis Elevation"
  Average S1 Selector/1 -> Cardiac Mechanical Systolic Axis Finder 3D/1, Max S1 P2P  Axis Finder 3D/1
  Selector/1 -> MATLAB Function/2(el_scg), Display1/1, Mechanical Axis Elevation/1  "Mech Axis Elevation"
  Max S1 P2P  Axis Finder 3D/1 -> Selector7/1, Selector6/1, Selector2/1, Selector3/1
  Selector1/1 -> Mechanical Axis Azimuth/1, Display3/1, MATLAB Function/3(az_scg)  "Mech Axis Azimuth"
  Selector6/1 -> MATLAB Function3/2(el_scg), Display7/1, Min S1 P2Pamp Axis Elevation/1  "Antimech Axis Elevation"
  Cardiac Mechanical Systolic Axis Finder 3D/1 -> Selector5/1, Selector4/1, Selector/1, Selector1/1
  SCGxyz Average Cycle/1(out_scgxyz_avgcycle) -> Average S1 Selector/1
  Selector5/1 -> MATLAB Function1/3(az_scg), Antimechanical Axis Azimuth/1, Display5/1  "Antimech Axis Azimuth"
  MATLAB Function2/1(projection) -> Fixed-Size Converter2/1
  Selector7/1 -> MATLAB Function3/3(az_scg), Min S1 P2Pamp Axis Azimuth/1, Display8/1  "Antimech Axis Azimuth"
  Selector3/1 -> Max S1 P2Pamp Axis Azimuth/1, Display6/1, MATLAB Function2/3(az_scg)  "Max S1 Axis Azimuth"
  MATLAB Function1/1(projection) -> Fixed-Size Converter1/1
  MATLAB Function/1(projection) -> Fixed-Size Converter/1
  Fixed-Size Converter/1 -> Mechanical Axis Projection/1
  Fixed-Size Converter1/1 -> Antimechanical Axis Projection/1
  Fixed-Size Converter2/1 -> Max S1 P2Pamp Axis Projection/1
  MATLAB Function3/1(projection) -> Fixed-Size Converter3/1
  Fixed-Size Converter3/1 -> Min S1 P2Pamp Axis Projection/1

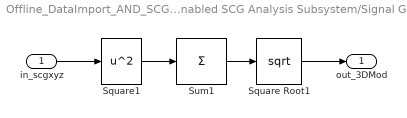
== system Offline_DataImport_AND_SCGAnalysis/SCG Analysis/Enabled SCG Analysis Subsystem/Signal Generation/3DMod Calculator ==
  in_scgxyz : Inport
  Square Root1 : Sqrt  SaturateOnIntegerOverflow=on
  Square1 : Math  Operator=square  SignedPower=on  SaturateOnIntegerOverflow=on
  Sum1 : Sum  Inputs=+  CollapseMode=Specified dimension  CollapseDim=2
  out_3DMod : Outport  VectorParamsAs1DForOutWhenUnconnected=off
  wires:
  Square1/1 -> Sum1/1
  Sum1/1 -> Square Root1/1
  in_scgxyz/1 -> Square1/1
  Square Root1/1 -> out_3DMod/1

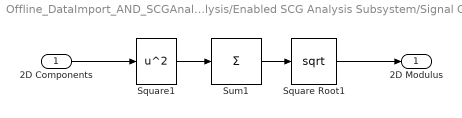
== system Offline_DataImport_AND_SCGAnalysis/SCG Analysis/Enabled SCG Analysis Subsystem/Signal Generation/2DMod Calculator/2DMod Calculator ==
  2D Components : Inport
  Square Root1 : Sqrt  SaturateOnIntegerOverflow=on
  Square1 : Math  Operator=square  SignedPower=on  SaturateOnIntegerOverflow=on
  Sum1 : Sum  Inputs=+  CollapseMode=Specified dimension  CollapseDim=2
  2D Modulus : Outport  VectorParamsAs1DForOutWhenUnconnected=off
  wires:
  Square1/1 -> Sum1/1
  Sum1/1 -> Square Root1/1
  2D Components/1 -> Square1/1
  Square Root1/1 -> 2D Modulus/1

== system Offline_DataImport_AND_SCGAnalysis/SCG Analysis/Enabled SCG Analysis Subsystem/Signal Generation/3D Projections/SCGxyz Average Cycle ==
  in_scgxyz : Inport
  Average SCGxyz Cycle Calculator : MATLAB Function  TreatAsAtomicUnit=on
  Constant : Constant  Value=analyses.ecg.R
  Fixed-Size Converter 2 : Selector  NumberOfDimensions=2  IndexOptions=Index vector (dialog),Index vector (dialog)  Indices=[1:min(analyses.ecg.RR)],[1:3]  OutputSizes=1,1
  out_scgxyz_avgcycle : Outport  VectorParamsAs1DForOutWhenUnconnected=off
  wires:
  in_scgxyz/1 -> Average SCGxyz Cycle Calculator/1(scgxyz)
  Constant/1 -> Average SCGxyz Cycle Calculator/2(r_pos)
  Average SCGxyz Cycle Calculator/1(scgxyz_avgcycle) -> Fixed-Size Converter 2/1
  Fixed-Size Converter 2/1 -> out_scgxyz_avgcycle/1

== matlab function Offline_DataImport_AND_SCGAnalysis/SCG Analysis/Enabled SCG Analysis Subsystem/Signal Generation/2D Mod Average Cycle/Average 2DMod Cycle Calculator ==
  data: signal input; r_pos input; avg_cycle output size=[min(analyses.ecg.RR) 1]
function avg_cycle  = slk_avg_cycle_calculator(signal, r_pos)
% Simulink function to return the average cycle of an arbitraty signal input.

% INPUTS:
% r_pos = index positions of the R peaks of the ecg.
% signal = arbitrary input signal.

% OUTPUT:
% avg_cycle = averaged cycle of arbitrary input signal.


% Calculating number of cycles to be considered in averaging
rr_min = min(diff(r_pos)); % Shortest cycle length - all the cycles will but cut down to this length.

if length(signal) > r_pos(end) + rr_min
    considered_cycles = length(r_pos);
else
    considered_cycles = length(r_pos) - 1;
end

signal_cycles = zeros(rr_min,considered_cycles);

fig_average_cycle = figure;

% Isolating and plotting each cycle
for i = 1:considered_cycles
    signal_cycles(:,i) = signal(r_pos(i):r_pos(i) + rr_min - 1,1);
    figure(fig_average_cycle); plot(signal_cycles(:,i),'b'); hold on
end

% Calculating average cycle
avg_cycle = mean(signal_cycles,2);

% Plotting the average cycle
figure(fig_average_cycle); plot(avg_cycle,'k','LineWidth',2); title('Average Cycle'); xlabel('Time (msec)'); ylabel('Acceleration (mg)'); box off;
title('2D Modulus')
end

== matlab function Offline_DataImport_AND_SCGAnalysis/SCG Analysis/Enabled SCG Analysis Subsystem/Signal Generation/3D Projections/MATLAB Function ==
  data: scg_xyz input; el_scg input; projection output size=[1 param_tot_samples]; az_scg input
function projection = slk_axis_projection(scg_xyz, el_scg, az_scg)

el_mat = el_scg;
az_mat = -1*az_scg;

[xhat_mat, yhat_mat, zhat_mat] = sph2cart(az_mat*pi/180,el_mat*pi/180,1);
% Converting to the SCG convention reference frame (this depends on the accelerometer and its placement orientation! - they should be such that they match the conventional SCG reference frame).
xhat_scg = xhat_mat;
yhat_scg = zhat_mat;
zhat_scg = -1*yhat_mat;

projection_axis = [xhat_scg yhat_scg zhat_scg];
    
projection = zeros(1,size(scg_xyz,1));
    
for i=1:size(scg_xyz,1)
    
    projection(i) = dot(scg_xyz(i,:),projection_axis);
    
end

figure;
ax = [0 0 0 0];

ax(1) = subplot(4,1,1); plot(scg_xyz(:,1),'b'); title('x'); box off; ylabel('Acceleration (mg)');
ax(2) = subplot(4,1,2); plot(scg_xyz(:,2),'b'); title('y'); box off; ylabel('Acceleration (mg)');
ax(3) = subplot(4,1,3); plot(scg_xyz(:,3),'b'); title('z'); box off; ylabel('Acceleration (mg)');
ax(4) = subplot(4,1,4); plot(projection,'g'); title('Mechanical Axis Projection'); box off; ylabel('Acceleration (mg)');
xlabel('Sample no.')
linkaxes(ax,'xy')
end

== matlab function Offline_DataImport_AND_SCGAnalysis/SCG Analysis/Enabled SCG Analysis Subsystem/Signal Generation/3D Mod Average Cycle/Average 3DMod Cycle Calculator ==
  data: signal input; r_pos input; avg_cycle output size=[min(analyses.ecg.RR) 1]
function avg_cycle  = slk_avg_cycle_calculator(signal, r_pos)
% Simulink function to return the average cycle of an arbitraty signal input.

% INPUTS:
% r_pos = index positions of the R peaks of the ecg.
% signal = arbitrary input signal.

% OUTPUT:
% avg_cycle = averaged cycle of arbitrary input signal.


% Calculating number of cycles to be considered in averaging
rr_min = min(diff(r_pos)); % Shortest cycle length - all the cycles will but cut down to this length.

if length(signal) > r_pos(end) + rr_min
    considered_cycles = length(r_pos);
else
    considered_cycles = length(r_pos) - 1;
end

signal_cycles = zeros(rr_min,considered_cycles);

fig_average_cycle = figure;

% Isolating and plotting each cycle
for i = 1:considered_cycles
    figure(fig_average_cycle);
    signal_cycles(:,i) = signal(r_pos(i):r_pos(i) + rr_min - 1,1);
    plot(signal_cycles(:,i),'b'); hold on
end

% Calculating average cycle
avg_cycle = mean(signal_cycles,2);

% Plotting the average cycle
plot(avg_cycle,'k','LineWidth',2); title('Average Cycle'); xlabel('Time (msec)'); ylabel('Acceleration (mg)'); box off;
title('3D Modulus')
end

== matlab function Offline_DataImport_AND_SCGAnalysis/SCG Analysis/Enabled SCG Analysis Subsystem/Signal Generation/3D Projections/SCGxyz Average Cycle/Average SCGxyz Cycle Calculator ==
  data: scgxyz input; r_pos input; scgxyz_avgcycle output size=[min(analyses.ecg.RR) 3]
function scgxyz_avgcycle  = slk_avg_scgxyz_cycle_calculator(scgxyz,r_pos)
% Simulink function to return the average x,y, and z cycles of the SCG.

% INPUTS:
% r_pos = index positions of the R peaks of the ecg.
% scgxyz = matrix of size [length_scg 3] with the (normally pre-processed) SCG
%          x,y, and z components. The first column corresponds to SCGx, the second
%          to SCGy and the third to SCGz.

% OUTPUT:
% avg_scg_xyz = matrix of size [min_rr 3] with the average SCG cycles of
%               the x,y, and z components. The first column corresponds to SCGx, the second
%               to SCGy and the third to SCGz 


% Calculating number of cycles to be considered in averaging (considered_cycles).
rr_min = min(diff(r_pos)); % Shortest cycle length - all the cycles will but cut down to this length.

if length(scgxyz) > r_pos(end) + rr_min
    considered_cycles = length(r_pos);
else
    considered_cycles = length(r_pos) - 1;
end

scg_x_cycles = zeros(rr_min,considered_cycles);
scg_y_cycles = zeros(rr_min,considered_cycles);
scg_z_cycles = zeros(rr_min,considered_cycles);

fig_scg_average_cycles = figure;

% Isolating and plotting each cycle
for i = 1:considered_cycles
    figure(fig_scg_average_cycles);
    scg_x_cycles(:,i) = scgxyz(r_pos(i):r_pos(i) + rr_min - 1,1);
    scg_y_cycles(:,i) = scgxyz(r_pos(i):r_pos(i) + rr_min - 1,2);
    scg_z_cycles(:,i) = scgxyz(r_pos(i):r_pos(i) + rr_min - 1,3);
    
    % Plotting
    subplot(3,1,1); plot(scg_x_cycles(:,i),'b'); hold on;
    subplot(3,1,2); plot(scg_y_cycles(:,i),'b'); hold on;
    subplot(3,1,3); plot(scg_z_cycles(:,i),'b'); hold on;
end

% Calculating average cycle
avg_scg_x = mean(scg_x_cycles,2);
avg_scg_y = mean(scg_y_cycles,2);
avg_scg_z = mean(scg_z_cycles,2);

% Plotting the average cycle
subplot(3,1,1); plot(avg_scg_x,'k','LineWidth',2); title('Average SCG x'); box off;
subplot(3,1,2); plot(avg_scg_y,'k','LineWidth',2); title('Average SCG y'); ylabel('Amplitude (mg)'); box off;
subplot(3,1,3); plot(avg_scg_z,'k','LineWidth',2); title('Average SCG z'); xlabel('Time (msec)'); box off;

scgxyz_avgcycle = [avg_scg_x avg_scg_y avg_scg_z];
end

== matlab function Offline_DataImport_AND_SCGAnalysis/SCG Analysis/Enabled SCG Analysis Subsystem/Signal Generation/3D Projections/MATLAB Function1 ==
  data: scg_xyz input; el_scg input; projection output size=[1 param_tot_samples]; az_scg input
function projection = slk_axis_projection(scg_xyz, el_scg, az_scg)

el_mat = el_scg;
az_mat = -1*az_scg;

[xhat_mat, yhat_mat, zhat_mat] = sph2cart(az_mat*pi/180,el_mat*pi/180,1);
% Converting to the SCG convention reference frame (this depends on the accelerometer and its placement orientation! - they should be such that they match the conventional SCG reference frame).
xhat_scg = xhat_mat;
yhat_scg = zhat_mat;
zhat_scg = -1*yhat_mat;

projection_axis = [xhat_scg yhat_scg zhat_scg];
    
projection = zeros(1,size(scg_xyz,1));
    
for i=1:size(scg_xyz,1)
    
    projection(i) = dot(scg_xyz(i,:),projection_axis);
    
end

figure;
ax = [0 0 0 0];

ax(1) = subplot(4,1,1); plot(scg_xyz(:,1),'b'); title('x'); box off; ylabel('Acceleration (mg)');
ax(2) = subplot(4,1,2); plot(scg_xyz(:,2),'b'); title('y'); box off; ylabel('Acceleration (mg)');
ax(3) = subplot(4,1,3); plot(scg_xyz(:,3),'b'); title('z'); box off; ylabel('Acceleration (mg)');
ax(4) = subplot(4,1,4); plot(projection,'r'); title('Antimechanical Axis Projection'); box off; ylabel('Acceleration (mg)');
xlabel('Sample no.')
linkaxes(ax,'xy')
end

== matlab function Offline_DataImport_AND_SCGAnalysis/SCG Analysis/Enabled SCG Analysis Subsystem/Signal Generation/3D Projections/MATLAB Function2 ==
  data: scg_xyz input; el_scg input; projection output size=[1 param_tot_samples]; az_scg input
function projection = slk_axis_projection(scg_xyz, el_scg, az_scg)

el_mat = el_scg;
az_mat = -1*az_scg;

[xhat_mat, yhat_mat, zhat_mat] = sph2cart(az_mat*pi/180,el_mat*pi/180,1);
% Converting to the SCG convention reference frame (this depends on the accelerometer and its placement orientation! - they should be such that they match the conventional SCG reference frame).
xhat_scg = xhat_mat;
yhat_scg = zhat_mat;
zhat_scg = -1*yhat_mat;

projection_axis = [xhat_scg yhat_scg zhat_scg];
    
projection = zeros(1,size(scg_xyz,1));
    
for i=1:size(scg_xyz,1)
    
    projection(i) = dot(scg_xyz(i,:),projection_axis);
    
end

figure;
ax = [0 0 0 0];

ax(1) = subplot(4,1,1); plot(scg_xyz(:,1),'b'); title('x'); box off; ylabel('Acceleration (mg)');
ax(2) = subplot(4,1,2); plot(scg_xyz(:,2),'b'); title('y'); box off; ylabel('Acceleration (mg)');
ax(3) = subplot(4,1,3); plot(scg_xyz(:,3),'b'); title('z'); box off; ylabel('Acceleration (mg)');
ax(4) = subplot(4,1,4); plot(projection,'g'); title('Max S1 P2P Axis Projection'); box off; ylabel('Acceleration (mg)');
xlabel('Sample no.')
linkaxes(ax,'xy')
end

== matlab function Offline_DataImport_AND_SCGAnalysis/SCG Analysis/Enabled SCG Analysis Subsystem/Signal Generation/3D Projections/MATLAB Function3 ==
  data: scg_xyz input; el_scg input; projection output size=[1 param_tot_samples]; az_scg input
function projection = slk_axis_projection(scg_xyz, el_scg, az_scg)

el_mat = el_scg;
az_mat = -1*az_scg;

[xhat_mat, yhat_mat, zhat_mat] = sph2cart(az_mat*pi/180,el_mat*pi/180,1);
% Converting to the SCG convention reference frame (this depends on the accelerometer and its placement orientation! - they should be such that they match the conventional SCG reference frame).
xhat_scg = xhat_mat;
yhat_scg = zhat_mat;
zhat_scg = -1*yhat_mat;

projection_axis = [xhat_scg yhat_scg zhat_scg];
    
projection = zeros(1,size(scg_xyz,1));
    
for i=1:size(scg_xyz,1)
    
    projection(i) = dot(scg_xyz(i,:),projection_axis);
    
end

figure;
ax = [0 0 0 0];

ax(1) = subplot(4,1,1); plot(scg_xyz(:,1),'b'); title('x'); box off; ylabel('Acceleration (mg)');
ax(2) = subplot(4,1,2); plot(scg_xyz(:,2),'b'); title('y'); box off; ylabel('Acceleration (mg)');
ax(3) = subplot(4,1,3); plot(scg_xyz(:,3),'b'); title('z'); box off; ylabel('Acceleration (mg)');
ax(4) = subplot(4,1,4); plot(projection,'r'); title('Min S1 P2P Axis Projection'); box off; ylabel('Acceleration (mg)');
xlabel('Sample no.')
linkaxes(ax,'xy')
end

== matlab function Offline_DataImport_AND_SCGAnalysis/SCG Analysis/Enabled SCG Analysis Subsystem/Anisotropy Characterization/Wrapped Average Diameter//Volume Calculator ==
  data: fs input; average_diameter_over_volume output; r_pos input; scg_xyz input
function average_diameter_over_volume = wrapped_anisotropy_calculator_average_diameter_over_volume(fs,r_pos,scg_xyz) 
average_diameter_over_volume=-1; % Pre-Initialization.
coder.extrinsic('anisotropy_calculator_average_diameter_over_volume');
average_diameter_over_volume = anisotropy_calculator_average_diameter_over_volume(fs,r_pos,scg_xyz); %%%
